simulink model "stable"  (R2022a)
settings: Solver=ode4  StartTime=0.0  StopTime=10.0  FixedStep=0.001  RelTol=1e-3
settings Model: Creator=kcx06  LastModifiedBy=kcx06

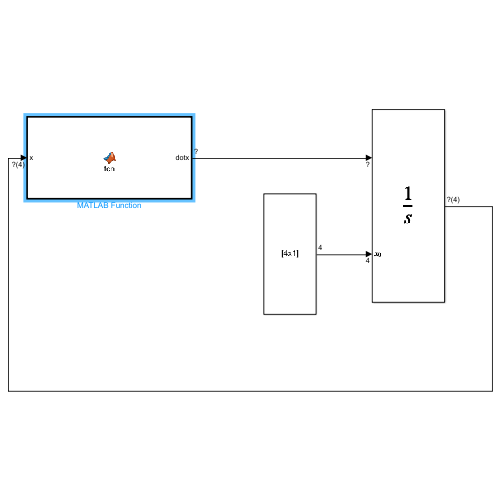
[thumbnail: Simulink's stored preview of the top-level diagram]
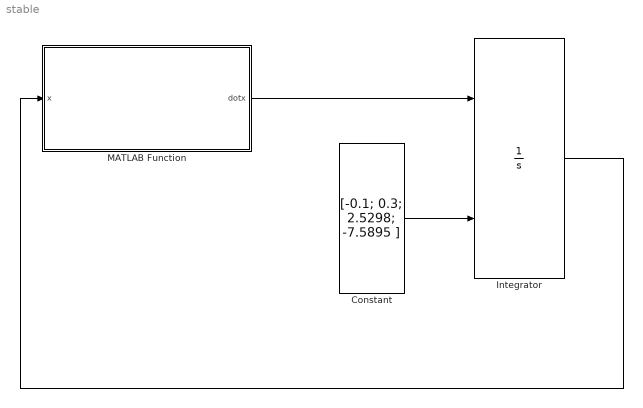
== system stable ==
  Constant : Constant  Value=[-0.1; 0.3; 2.5298; -7.5895 ]
  Integrator : Integrator  InitialConditionSource=external
  MATLAB Function : MATLAB Function  TreatAsAtomicUnit=on
  wires:
  MATLAB Function/1(dotx) -> Integrator/1
  Constant/1 -> Integrator/2
  Integrator/1 -> MATLAB Function/1(x)

== matlab function stable/MATLAB Function ==
  data: x input; dotx output
function dotx = fcn(x)
r_ss = -24;
A = [0 r_ss 0 -1;
     -r_ss 0 1 0;
     0 0 0 -0.5*r_ss;
     0 0 0.5*r_ss 0];
dotx = A*x;
